simulink model "architecture"  (R2021b)
settings: Solver=FixedStepAuto  StartTime=0.0  StopTime=10.0  FixedStep=sampleTime.digital  RelTol=1e-3
libraries: EMACE_APP x6, AEMACE10_IN x1, AEMACE10_INSTRUMENTATION x1, AEMACE10_OUT x1, AEMACE8_IN x1, AEMACE8_INSTRUMENTATION x1, AEMACE8_OUT x1, SEMACE1_IN x1, SEMACE1_INSTRUMENTATION x1, SEMACE1_OUT x1, SEMACE2_IN x1, SEMACE2_INSTRUMENTATION x1
settings Model: DataDictionary=targetDD.sldd  Creator=ACH  LastModifiedBy=ACH

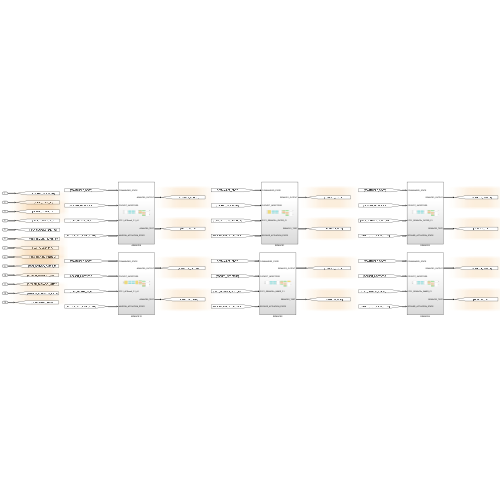
[thumbnail: Simulink's stored preview of the top-level diagram]
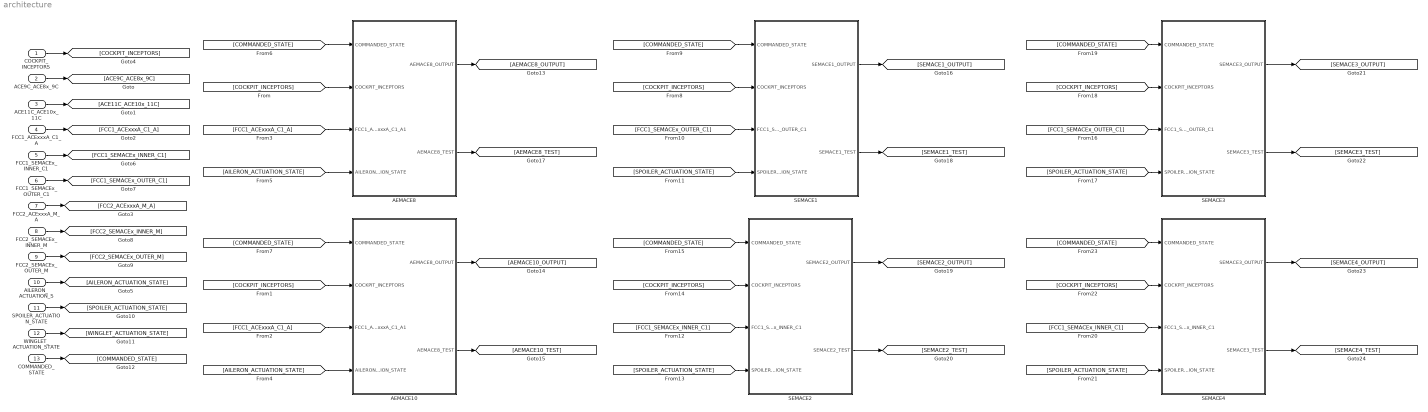
== system architecture ==
  COCKPIT_INCEPTORS : Inport  OutDataTypeStr=Bus: COCKPIT_INCEPTORS
  ACE9C_ACE8x_9C : Inport  Port=2  OutDataTypeStr=Bus: ACE9C_ACE8x_9C
  ACE11C_ACE10x_11C : Inport  Port=3  OutDataTypeStr=Bus: ACE11C_ACE10x_11C
  FCC1_ACExxxA_C1_A : Inport  Port=4  OutDataTypeStr=Bus: FCC1_ACExxxA_C1_A
  FCC1_SEMACEx_INNER_C1 : Inport  Port=5  OutDataTypeStr=Bus: FCC1_SEMACEx_INNER_C1
  FCC1_SEMACEx_OUTER_C1 : Inport  Port=6  OutDataTypeStr=Bus: FCC1_SEMACEx_OUTER_C1
  FCC2_ACExxxA_M_A : Inport  Port=7  OutDataTypeStr=Bus: FCC2_ACExxxA_M_A
  FCC2_SEMACEx_INNER_M : Inport  Port=8  OutDataTypeStr=Bus: FCC2_SEMACEx_INNER_M
  FCC2_SEMACEx_OUTER_M : Inport  Port=9  OutDataTypeStr=Bus: FCC2_SEMACEx_OUTER_M
  AILERON_ACTUATION_S : Inport  Port=10  OutDataTypeStr=Bus: AILERON_ACTUATION_STATE
  SPOILER_ACTUATION_STATE : Inport  Port=11  OutDataTypeStr=Bus: SPOILER_ACTUATION_STATE
  WINGLET_ACTUATION_STATE : Inport  Port=12  OutDataTypeStr=Bus: WINGLET_ACTUATION_STATE
  COMMANDED_STATE : Inport  Port=13  OutDataTypeStr=Bus: COMMANDED_STATE
  AEMACE10 : Subsystem
  AEMACE8 : Subsystem
  SEMACE1 : Subsystem
  SEMACE2 : Subsystem
  SEMACE3 : Subsystem
  SEMACE4 : Subsystem
  wires:
  ACE9C_ACE8x_9C/1 -> [ACE9C_ACE8x_9C]
  ACE11C_ACE10x_11C/1 -> [ACE11C_ACE10x_11C]
  FCC1_ACExxxA_C1_A/1 -> [FCC1_ACExxxA_C1_A]
  FCC2_ACExxxA_M_A/1 -> [FCC2_ACExxxA_M_A]
  COCKPIT_INCEPTORS/1 -> [COCKPIT_INCEPTORS]
  AILERON_ACTUATION_S/1 -> [AILERON_ACTUATION_STATE]
  FCC1_SEMACEx_INNER_C1/1 -> [FCC1_SEMACEx_INNER_C1]
  FCC1_SEMACEx_OUTER_C1/1 -> [FCC1_SEMACEx_OUTER_C1]
  FCC2_SEMACEx_INNER_M/1 -> [FCC2_SEMACEx_INNER_M]
  FCC2_SEMACEx_OUTER_M/1 -> [FCC2_SEMACEx_OUTER_M]
  SPOILER_ACTUATION_STATE/1 -> [SPOILER_ACTUATION_STATE]
  WINGLET_ACTUATION_STATE/1 -> [WINGLET_ACTUATION_STATE]
  COMMANDED_STATE/1 -> [COMMANDED_STATE]
  [COMMANDED_STATE] -> AEMACE8/1(COMMANDED_STATE)
  [COCKPIT_INCEPTORS] -> AEMACE8/2(COCKPIT_INCEPTORS)
  [FCC1_ACExxxA_C1_A] -> AEMACE8/3(FCC1_ACExxxA_C1_A1)
  [AILERON_ACTUATION_STATE] -> AEMACE8/4(AILERON_ACTUATION_STATE)
  AEMACE8/2(AEMACE8_TEST) -> [AEMACE8_TEST]
  AEMACE8/1(AEMACE8_OUTPUT) -> [AEMACE8_OUTPUT]
  [COMMANDED_STATE] -> AEMACE10/1(COMMANDED_STATE)
  [COCKPIT_INCEPTORS] -> AEMACE10/2(COCKPIT_INCEPTORS)
  [FCC1_ACExxxA_C1_A] -> AEMACE10/3(FCC1_ACExxxA_C1_A1)
  [AILERON_ACTUATION_STATE] -> AEMACE10/4(AILERON_ACTUATION_STATE)
  AEMACE10/1(AEMACE8_OUTPUT) -> [AEMACE10_OUTPUT]
  AEMACE10/2(AEMACE8_TEST) -> [AEMACE10_TEST]
  [COCKPIT_INCEPTORS] -> SEMACE1/2(COCKPIT_INCEPTORS)
  [COMMANDED_STATE] -> SEMACE1/1(COMMANDED_STATE)
  [FCC1_SEMACEx_OUTER_C1] -> SEMACE1/3(FCC1_SEMACEx_OUTER_C1)
  [SPOILER_ACTUATION_STATE] -> SEMACE1/4(SPOILER_ACTUATION_STATE)
  SEMACE1/1(SEMACE1_OUTPUT) -> [SEMACE1_OUTPUT]
  SEMACE1/2(SEMACE1_TEST) -> [SEMACE1_TEST]
  [SPOILER_ACTUATION_STATE] -> SEMACE2/4(SPOILER_ACTUATION_STATE)
  [COMMANDED_STATE] -> SEMACE2/1(COMMANDED_STATE)
  [COCKPIT_INCEPTORS] -> SEMACE2/2(COCKPIT_INCEPTORS)
  [FCC1_SEMACEx_INNER_C1] -> SEMACE2/3(FCC1_SEMACEx_INNER_C1)
  SEMACE2/1(SEMACE2_OUTPUT) -> [SEMACE2_OUTPUT]
  SEMACE2/2(SEMACE2_TEST) -> [SEMACE2_TEST]
  [COMMANDED_STATE] -> SEMACE3/1(COMMANDED_STATE)
  [COCKPIT_INCEPTORS] -> SEMACE3/2(COCKPIT_INCEPTORS)
  [FCC1_SEMACEx_OUTER_C1] -> SEMACE3/3(FCC1_SEMACEx_OUTER_C1)
  [SPOILER_ACTUATION_STATE] -> SEMACE3/4(SPOILER_ACTUATION_STATE)
  SEMACE3/1(SEMACE3_OUTPUT) -> [SEMACE3_OUTPUT]
  SEMACE3/2(SEMACE3_TEST) -> [SEMACE3_TEST]
  [COMMANDED_STATE] -> SEMACE4/1(COMMANDED_STATE)
  [COCKPIT_INCEPTORS] -> SEMACE4/2(COCKPIT_INCEPTORS)
  [FCC1_SEMACEx_INNER_C1] -> SEMACE4/3(FCC1_SEMACEx_INNER_C1)
  [SPOILER_ACTUATION_STATE] -> SEMACE4/4(SPOILER_ACTUATION_STATE)
  SEMACE4/1(SEMACE3_OUTPUT) -> [SEMACE4_OUTPUT]
  SEMACE4/2(SEMACE3_TEST) -> [SEMACE4_TEST]

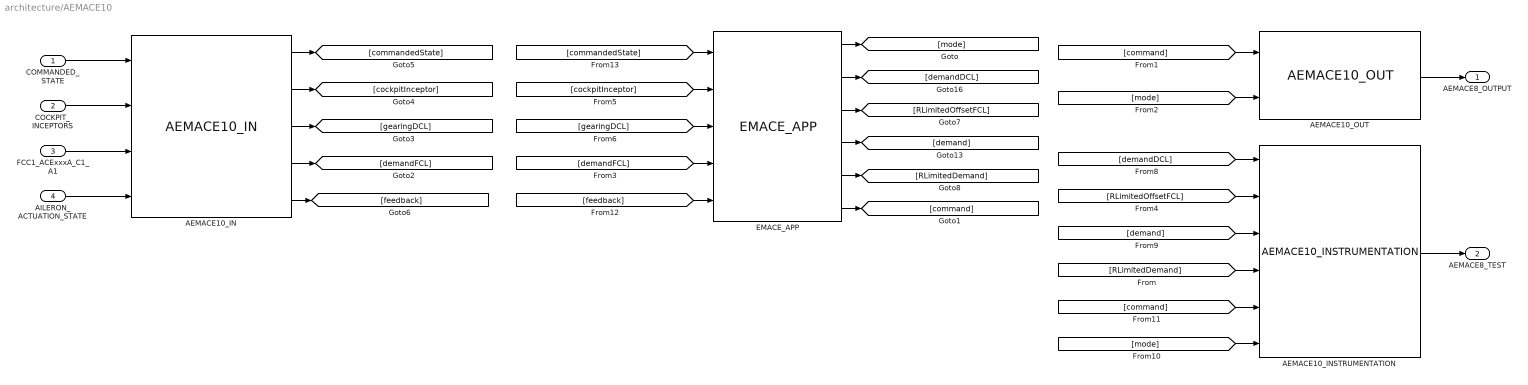
== system architecture/AEMACE10 ==
  COMMANDED_STATE : Inport
  COCKPIT_INCEPTORS : Inport  Port=2
  FCC1_ACExxxA_C1_A1 : Inport  Port=3
  AILERON_ACTUATION_STATE : Inport  Port=4
  AEMACE10_IN : AEMACE10_IN/AEMACE10_IN  SystemSampleTime=-1  VariantActivationTime=update diagram  Latency=0  AutoFrameSizeCalculation=off
  AEMACE10_INSTRUMENTATION : AEMACE10_INSTRUMENTATION/AEMACE10_INSTRUMENTATION  SystemSampleTime=-1  VariantActivationTime=update diagram  Latency=0  AutoFrameSizeCalculation=off
  AEMACE10_OUT : AEMACE10_OUT/AEMACE10_OUT  SystemSampleTime=-1  VariantActivationTime=update diagram  Latency=0  AutoFrameSizeCalculation=off
  EMACE_APP : EMACE_APP/EMACE_APP  SystemSampleTime=-1  VariantActivationTime=update diagram  Latency=0  AutoFrameSizeCalculation=off
      link override From10: GotoTag=command
  AEMACE8_OUTPUT : Outport
  AEMACE8_TEST : Outport  Port=2
  wires:
  COMMANDED_STATE/1 -> AEMACE10_IN/1
  COCKPIT_INCEPTORS/1 -> AEMACE10_IN/2
  FCC1_ACExxxA_C1_A1/1 -> AEMACE10_IN/3
  AILERON_ACTUATION_STATE/1 -> AEMACE10_IN/4
  AEMACE10_IN/1 -> [commandedState]
  AEMACE10_IN/2 -> [cockpitInceptor]
  AEMACE10_IN/3 -> [gearingDCL]
  AEMACE10_IN/4 -> [demandFCL]
  AEMACE10_IN/5 -> [feedback]
  [command] -> AEMACE10_OUT/1
  [mode] -> AEMACE10_OUT/2
  AEMACE10_OUT/1 -> AEMACE8_OUTPUT/1
  [demandDCL] -> AEMACE10_INSTRUMENTATION/1
  AEMACE10_INSTRUMENTATION/1 -> AEMACE8_TEST/1
  [commandedState] -> EMACE_APP/1
  [cockpitInceptor] -> EMACE_APP/2
  [gearingDCL] -> EMACE_APP/3
  [demandFCL] -> EMACE_APP/4
  [feedback] -> EMACE_APP/5
  EMACE_APP/1 -> [mode]
  EMACE_APP/2 -> [demandDCL]
  EMACE_APP/6 -> [command]
  EMACE_APP/4 -> [demand]
  EMACE_APP/3 -> [RLimitedOffsetFCL]
  EMACE_APP/5 -> [RLimitedDemand]
  [mode] -> AEMACE10_INSTRUMENTATION/6
  [command] -> AEMACE10_INSTRUMENTATION/5
  [RLimitedDemand] -> AEMACE10_INSTRUMENTATION/4
  [demand] -> AEMACE10_INSTRUMENTATION/3
  [RLimitedOffsetFCL] -> AEMACE10_INSTRUMENTATION/2

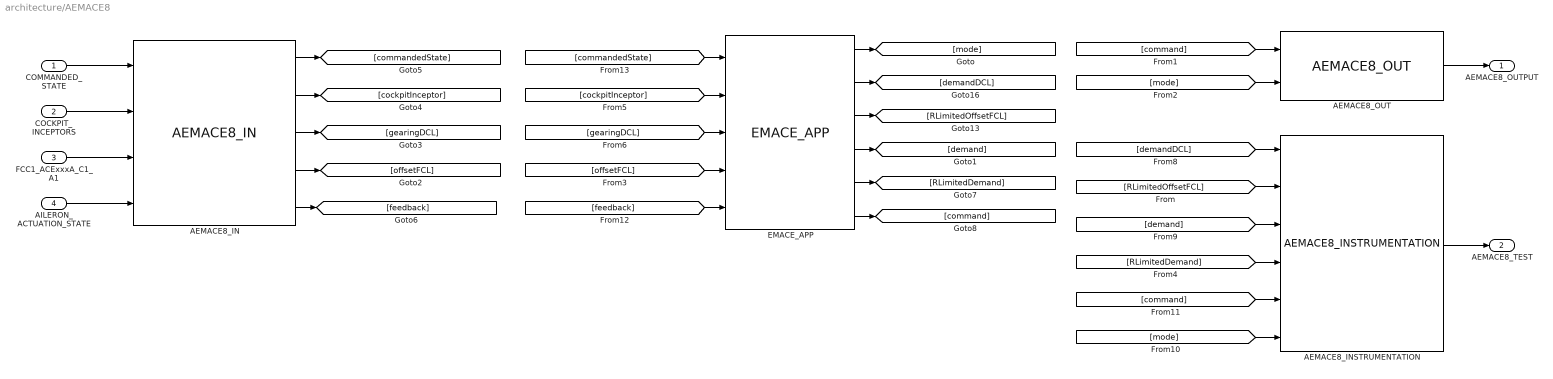
== system architecture/AEMACE8 ==
  COMMANDED_STATE : Inport
  COCKPIT_INCEPTORS : Inport  Port=2
  FCC1_ACExxxA_C1_A1 : Inport  Port=3
  AILERON_ACTUATION_STATE : Inport  Port=4
  AEMACE8_IN : AEMACE8_IN/AEMACE8_IN  SystemSampleTime=-1  VariantActivationTime=update diagram  Latency=0  AutoFrameSizeCalculation=off
      link override Rate Limiter: RisingSlewLimit=dataAEMACE.rateLimiterGearing  FallingSlewLimit=-dataAEMACE.rateLimiterGearing
  AEMACE8_INSTRUMENTATION : AEMACE8_INSTRUMENTATION/AEMACE8_INSTRUMENTATION  SystemSampleTime=-1  VariantActivationTime=update diagram  Latency=0  AutoFrameSizeCalculation=off
  AEMACE8_OUT : AEMACE8_OUT/AEMACE8_OUT  SystemSampleTime=-1  VariantActivationTime=update diagram  Latency=0  AutoFrameSizeCalculation=off
  EMACE_APP : EMACE_APP/EMACE_APP  SystemSampleTime=-1  VariantActivationTime=update diagram  Latency=0  AutoFrameSizeCalculation=off
  AEMACE8_OUTPUT : Outport
  AEMACE8_TEST : Outport  Port=2
  wires:
  COMMANDED_STATE/1 -> AEMACE8_IN/1
  COCKPIT_INCEPTORS/1 -> AEMACE8_IN/2
  FCC1_ACExxxA_C1_A1/1 -> AEMACE8_IN/3
  AILERON_ACTUATION_STATE/1 -> AEMACE8_IN/4
  AEMACE8_IN/1 -> [commandedState]
  AEMACE8_IN/2 -> [cockpitInceptor]
  AEMACE8_IN/3 -> [gearingDCL]
  AEMACE8_IN/4 -> [offsetFCL]
  AEMACE8_IN/5 -> [feedback]
  [command] -> AEMACE8_OUT/1
  [mode] -> AEMACE8_OUT/2
  AEMACE8_OUT/1 -> AEMACE8_OUTPUT/1
  [demandDCL] -> AEMACE8_INSTRUMENTATION/1
  AEMACE8_INSTRUMENTATION/1 -> AEMACE8_TEST/1
  [commandedState] -> EMACE_APP/1
  [cockpitInceptor] -> EMACE_APP/2
  [gearingDCL] -> EMACE_APP/3
  [offsetFCL] -> EMACE_APP/4
  [feedback] -> EMACE_APP/5
  EMACE_APP/1 -> [mode]
  EMACE_APP/2 -> [demandDCL]
  EMACE_APP/3 -> [RLimitedOffsetFCL]
  EMACE_APP/4 -> [demand]
  EMACE_APP/5 -> [RLimitedDemand]
  EMACE_APP/6 -> [command]
  [RLimitedOffsetFCL] -> AEMACE8_INSTRUMENTATION/2
  [demand] -> AEMACE8_INSTRUMENTATION/3
  [RLimitedDemand] -> AEMACE8_INSTRUMENTATION/4
  [command] -> AEMACE8_INSTRUMENTATION/5
  [mode] -> AEMACE8_INSTRUMENTATION/6

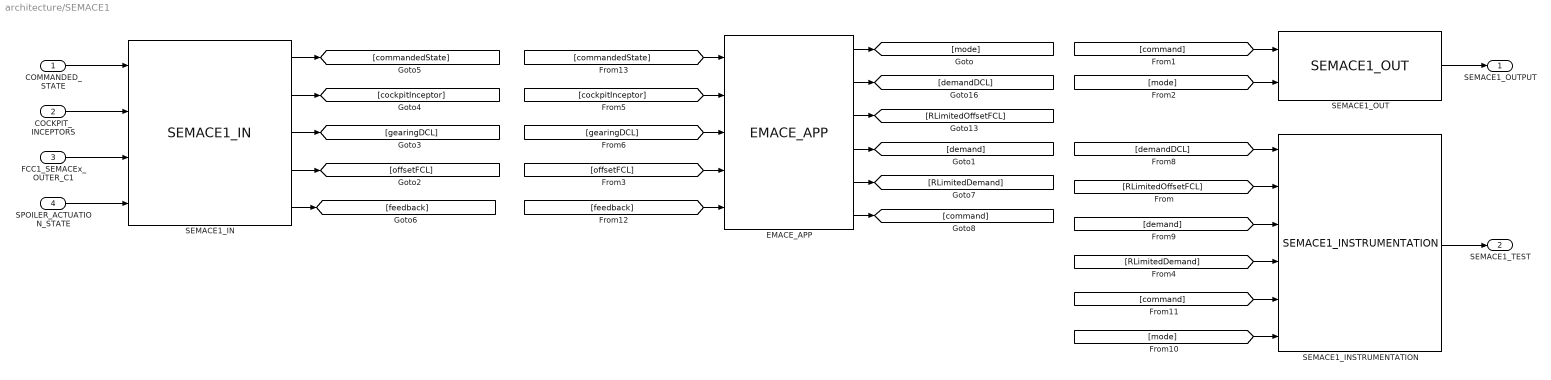
== system architecture/SEMACE1 ==
  COMMANDED_STATE : Inport
  COCKPIT_INCEPTORS : Inport  Port=2
  FCC1_SEMACEx_OUTER_C1 : Inport  Port=3  OutDataTypeStr=Bus: FCC1_SEMACEx_OUTER_C1
  SPOILER_ACTUATION_STATE : Inport  Port=4  OutDataTypeStr=Bus: SPOILER_ACTUATION_STATE
  EMACE_APP : EMACE_APP/EMACE_APP  SystemSampleTime=-1  VariantActivationTime=update diagram  Latency=0  AutoFrameSizeCalculation=off
  SEMACE1_IN : SEMACE1_IN/SEMACE1_IN  SystemSampleTime=-1  VariantActivationTime=update diagram  Latency=0  AutoFrameSizeCalculation=off
  SEMACE1_INSTRUMENTATION : SEMACE1_INSTRUMENTATION/SEMACE1_INSTRUMENTATION  SystemSampleTime=-1  VariantActivationTime=update diagram  Latency=0  AutoFrameSizeCalculation=off
  SEMACE1_OUT : SEMACE1_OUT/SEMACE1_OUT  SystemSampleTime=-1  VariantActivationTime=update diagram  Latency=0  AutoFrameSizeCalculation=off
  SEMACE1_OUTPUT : Outport
  SEMACE1_TEST : Outport  Port=2
  wires:
  COMMANDED_STATE/1 -> SEMACE1_IN/1
  COCKPIT_INCEPTORS/1 -> SEMACE1_IN/2
  FCC1_SEMACEx_OUTER_C1/1 -> SEMACE1_IN/3
  SPOILER_ACTUATION_STATE/1 -> SEMACE1_IN/4
  SEMACE1_IN/1 -> [commandedState]
  SEMACE1_IN/2 -> [cockpitInceptor]
  SEMACE1_IN/3 -> [gearingDCL]
  SEMACE1_IN/4 -> [offsetFCL]
  SEMACE1_IN/5 -> [feedback]
  [command] -> SEMACE1_OUT/1
  [mode] -> SEMACE1_OUT/2
  SEMACE1_OUT/1 -> SEMACE1_OUTPUT/1
  [demandDCL] -> SEMACE1_INSTRUMENTATION/1
  SEMACE1_INSTRUMENTATION/1 -> SEMACE1_TEST/1
  [commandedState] -> EMACE_APP/1
  [cockpitInceptor] -> EMACE_APP/2
  [gearingDCL] -> EMACE_APP/3
  [offsetFCL] -> EMACE_APP/4
  [feedback] -> EMACE_APP/5
  EMACE_APP/1 -> [mode]
  EMACE_APP/2 -> [demandDCL]
  EMACE_APP/3 -> [RLimitedOffsetFCL]
  EMACE_APP/4 -> [demand]
  EMACE_APP/5 -> [RLimitedDemand]
  EMACE_APP/6 -> [command]
  [RLimitedOffsetFCL] -> SEMACE1_INSTRUMENTATION/2
  [demand] -> SEMACE1_INSTRUMENTATION/3
  [RLimitedDemand] -> SEMACE1_INSTRUMENTATION/4
  [command] -> SEMACE1_INSTRUMENTATION/5
  [mode] -> SEMACE1_INSTRUMENTATION/6

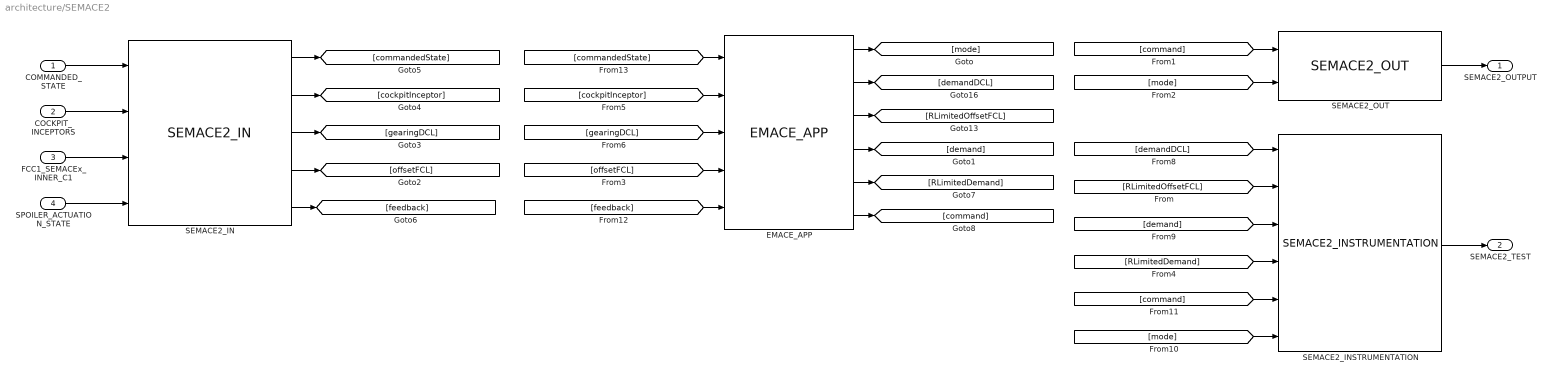
== system architecture/SEMACE2 ==
  COMMANDED_STATE : Inport
  COCKPIT_INCEPTORS : Inport  Port=2
  FCC1_SEMACEx_INNER_C1 : Inport  Port=3  OutDataTypeStr=Bus: FCC1_SEMACEx_INNER_C1
  SPOILER_ACTUATION_STATE : Inport  Port=4  OutDataTypeStr=Bus: SPOILER_ACTUATION_STATE
  EMACE_APP : EMACE_APP/EMACE_APP  SystemSampleTime=-1  VariantActivationTime=update diagram  Latency=0  AutoFrameSizeCalculation=off
  SEMACE2_IN : SEMACE2_IN/SEMACE2_IN  SystemSampleTime=-1  VariantActivationTime=update diagram  Latency=0  AutoFrameSizeCalculation=off
  SEMACE2_INSTRUMENTATION : SEMACE2_INSTRUMENTATION/SEMACE2_INSTRUMENTATION  SystemSampleTime=-1  VariantActivationTime=update diagram  Latency=0  AutoFrameSizeCalculation=off
  SEMACE2_OUT : SEMACE2_OUT/SEMACE2_OUT  SystemSampleTime=-1  VariantActivationTime=update diagram  Latency=0  AutoFrameSizeCalculation=off
  SEMACE2_OUTPUT : Outport
  SEMACE2_TEST : Outport  Port=2
  wires:
  [mode] -> SEMACE2_INSTRUMENTATION/6
  [command] -> SEMACE2_INSTRUMENTATION/5
  [RLimitedDemand] -> SEMACE2_INSTRUMENTATION/4
  [demand] -> SEMACE2_INSTRUMENTATION/3
  [RLimitedOffsetFCL] -> SEMACE2_INSTRUMENTATION/2
  EMACE_APP/6 -> [command]
  EMACE_APP/5 -> [RLimitedDemand]
  EMACE_APP/4 -> [demand]
  EMACE_APP/3 -> [RLimitedOffsetFCL]
  EMACE_APP/2 -> [demandDCL]
  EMACE_APP/1 -> [mode]
  [feedback] -> EMACE_APP/5
  [offsetFCL] -> EMACE_APP/4
  [gearingDCL] -> EMACE_APP/3
  [cockpitInceptor] -> EMACE_APP/2
  [commandedState] -> EMACE_APP/1
  SEMACE2_INSTRUMENTATION/1 -> SEMACE2_TEST/1
  [demandDCL] -> SEMACE2_INSTRUMENTATION/1
  SEMACE2_OUT/1 -> SEMACE2_OUTPUT/1
  [mode] -> SEMACE2_OUT/2
  [command] -> SEMACE2_OUT/1
  SEMACE2_IN/5 -> [feedback]
  SEMACE2_IN/4 -> [offsetFCL]
  SEMACE2_IN/3 -> [gearingDCL]
  SEMACE2_IN/2 -> [cockpitInceptor]
  SEMACE2_IN/1 -> [commandedState]
  SPOILER_ACTUATION_STATE/1 -> SEMACE2_IN/4
  FCC1_SEMACEx_INNER_C1/1 -> SEMACE2_IN/3
  COCKPIT_INCEPTORS/1 -> SEMACE2_IN/2
  COMMANDED_STATE/1 -> SEMACE2_IN/1

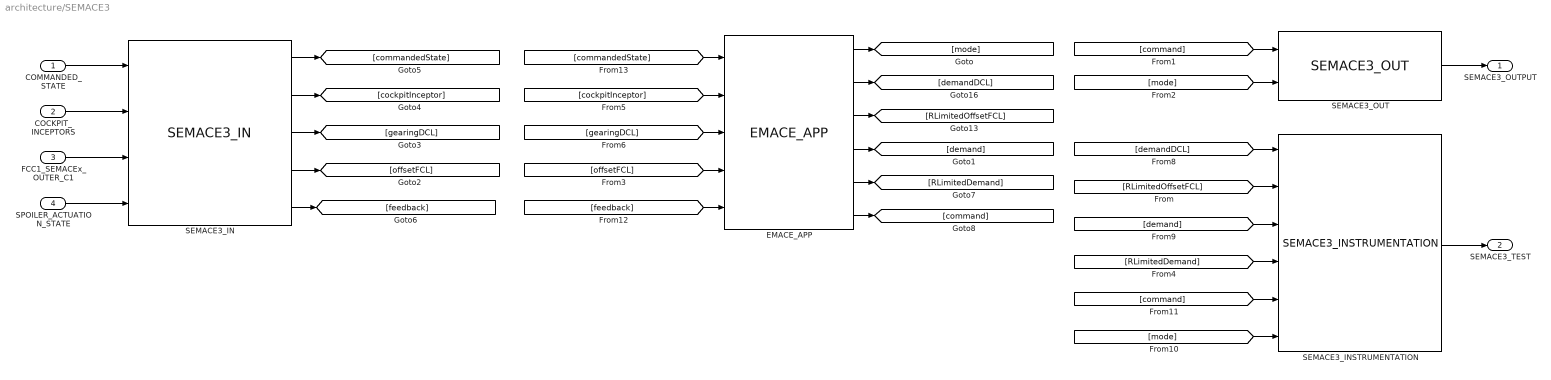
== system architecture/SEMACE3 ==
  COMMANDED_STATE : Inport
  COCKPIT_INCEPTORS : Inport  Port=2
  FCC1_SEMACEx_OUTER_C1 : Inport  Port=3  OutDataTypeStr=Bus: FCC1_SEMACEx_OUTER_C1
  SPOILER_ACTUATION_STATE : Inport  Port=4  OutDataTypeStr=Bus: SPOILER_ACTUATION_STATE
  EMACE_APP : EMACE_APP/EMACE_APP  SystemSampleTime=-1  VariantActivationTime=update diagram  Latency=0  AutoFrameSizeCalculation=off
  SEMACE3_IN : SEMACE3_IN/SEMACE3_IN  SystemSampleTime=-1  VariantActivationTime=update diagram  Latency=0  AutoFrameSizeCalculation=off
  SEMACE3_INSTRUMENTATION : SEMACE3_INSTRUMENTATION/SEMACE3_INSTRUMENTATION  SystemSampleTime=-1  VariantActivationTime=update diagram  Latency=0  AutoFrameSizeCalculation=off
  SEMACE3_OUT : SEMACE3_OUT/SEMACE3_OUT  SystemSampleTime=-1  VariantActivationTime=update diagram  Latency=0  AutoFrameSizeCalculation=off
  SEMACE3_OUTPUT : Outport
  SEMACE3_TEST : Outport  Port=2
  wires:
  [mode] -> SEMACE3_INSTRUMENTATION/6
  [command] -> SEMACE3_INSTRUMENTATION/5
  [RLimitedDemand] -> SEMACE3_INSTRUMENTATION/4
  [demand] -> SEMACE3_INSTRUMENTATION/3
  [RLimitedOffsetFCL] -> SEMACE3_INSTRUMENTATION/2
  EMACE_APP/6 -> [command]
  EMACE_APP/5 -> [RLimitedDemand]
  EMACE_APP/4 -> [demand]
  EMACE_APP/3 -> [RLimitedOffsetFCL]
  EMACE_APP/2 -> [demandDCL]
  EMACE_APP/1 -> [mode]
  [feedback] -> EMACE_APP/5
  [offsetFCL] -> EMACE_APP/4
  [gearingDCL] -> EMACE_APP/3
  [cockpitInceptor] -> EMACE_APP/2
  [commandedState] -> EMACE_APP/1
  SEMACE3_INSTRUMENTATION/1 -> SEMACE3_TEST/1
  [demandDCL] -> SEMACE3_INSTRUMENTATION/1
  SEMACE3_OUT/1 -> SEMACE3_OUTPUT/1
  [mode] -> SEMACE3_OUT/2
  [command] -> SEMACE3_OUT/1
  SEMACE3_IN/5 -> [feedback]
  SEMACE3_IN/4 -> [offsetFCL]
  SEMACE3_IN/3 -> [gearingDCL]
  SEMACE3_IN/2 -> [cockpitInceptor]
  SEMACE3_IN/1 -> [commandedState]
  SPOILER_ACTUATION_STATE/1 -> SEMACE3_IN/4
  FCC1_SEMACEx_OUTER_C1/1 -> SEMACE3_IN/3
  COCKPIT_INCEPTORS/1 -> SEMACE3_IN/2
  COMMANDED_STATE/1 -> SEMACE3_IN/1

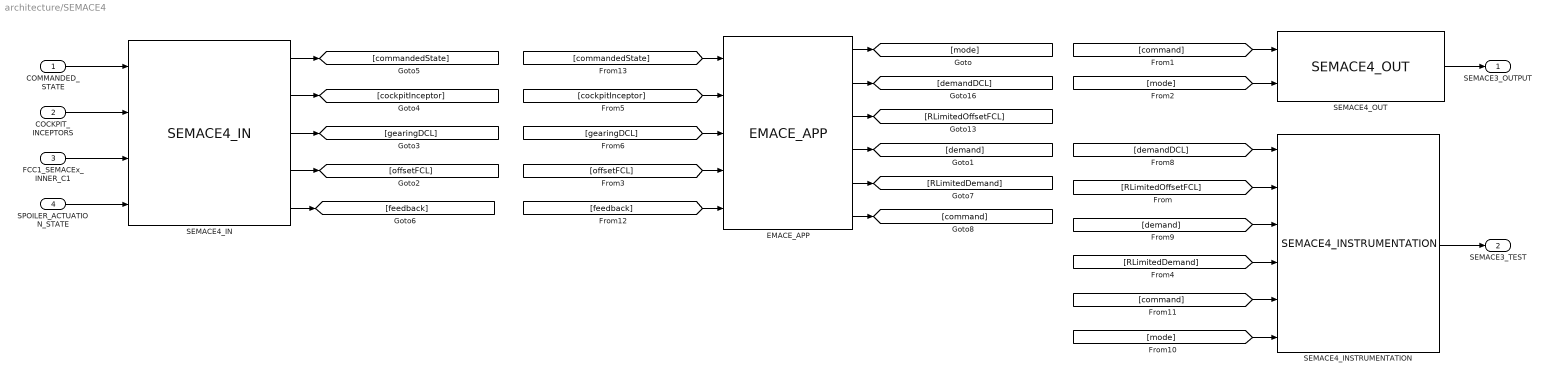
== system architecture/SEMACE4 ==
  COMMANDED_STATE : Inport
  COCKPIT_INCEPTORS : Inport  Port=2
  FCC1_SEMACEx_INNER_C1 : Inport  Port=3  OutDataTypeStr=Bus: FCC1_SEMACEx_INNER_C1
  SPOILER_ACTUATION_STATE : Inport  Port=4  OutDataTypeStr=Bus: SPOILER_ACTUATION_STATE
  EMACE_APP : EMACE_APP/EMACE_APP  SystemSampleTime=-1  VariantActivationTime=update diagram  Latency=0  AutoFrameSizeCalculation=off
  SEMACE4_IN : SEMACE4_IN/SEMACE4_IN  SystemSampleTime=-1  VariantActivationTime=update diagram  Latency=0  AutoFrameSizeCalculation=off
  SEMACE4_INSTRUMENTATION : SEMACE4_INSTRUMENTATION/SEMACE4_INSTRUMENTATION  SystemSampleTime=-1  VariantActivationTime=update diagram  Latency=0  AutoFrameSizeCalculation=off
  SEMACE4_OUT : SEMACE4_OUT/SEMACE4_OUT  SystemSampleTime=-1  VariantActivationTime=update diagram  Latency=0  AutoFrameSizeCalculation=off
  SEMACE3_OUTPUT : Outport
  SEMACE3_TEST : Outport  Port=2
  wires:
  COMMANDED_STATE/1 -> SEMACE4_IN/1
  COCKPIT_INCEPTORS/1 -> SEMACE4_IN/2
  FCC1_SEMACEx_INNER_C1/1 -> SEMACE4_IN/3
  SPOILER_ACTUATION_STATE/1 -> SEMACE4_IN/4
  SEMACE4_IN/1 -> [commandedState]
  SEMACE4_IN/2 -> [cockpitInceptor]
  SEMACE4_IN/3 -> [gearingDCL]
  SEMACE4_IN/4 -> [offsetFCL]
  SEMACE4_IN/5 -> [feedback]
  [command] -> SEMACE4_OUT/1
  [mode] -> SEMACE4_OUT/2
  SEMACE4_OUT/1 -> SEMACE3_OUTPUT/1
  [demandDCL] -> SEMACE4_INSTRUMENTATION/1
  SEMACE4_INSTRUMENTATION/1 -> SEMACE3_TEST/1
  [commandedState] -> EMACE_APP/1
  [cockpitInceptor] -> EMACE_APP/2
  [gearingDCL] -> EMACE_APP/3
  [offsetFCL] -> EMACE_APP/4
  [feedback] -> EMACE_APP/5
  EMACE_APP/1 -> [mode]
  EMACE_APP/2 -> [demandDCL]
  EMACE_APP/3 -> [RLimitedOffsetFCL]
  EMACE_APP/4 -> [demand]
  EMACE_APP/5 -> [RLimitedDemand]
  EMACE_APP/6 -> [command]
  [RLimitedOffsetFCL] -> SEMACE4_INSTRUMENTATION/2
  [demand] -> SEMACE4_INSTRUMENTATION/3
  [RLimitedDemand] -> SEMACE4_INSTRUMENTATION/4
  [command] -> SEMACE4_INSTRUMENTATION/5
  [mode] -> SEMACE4_INSTRUMENTATION/6
